simulink library "mag_vec_lib"  (R2016b)
settings: Solver=VariableStepAuto  StartTime=0.0  StopTime=10.0  RelTol=1e-3
undefined symbols (not defined in the file or in its folder): Earth, fsw_params, WGS84
libraries: aerolibtransform2 x2, dspmathops x1, aerolibgravity2 x1, YMDHMS_2_dec_year x1
settings Model: Creator=Taylor  LastModifiedBy=Taylor

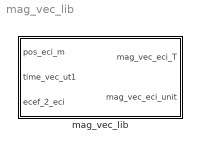
== system mag_vec_lib ==
  mag_vec_lib : Subsystem

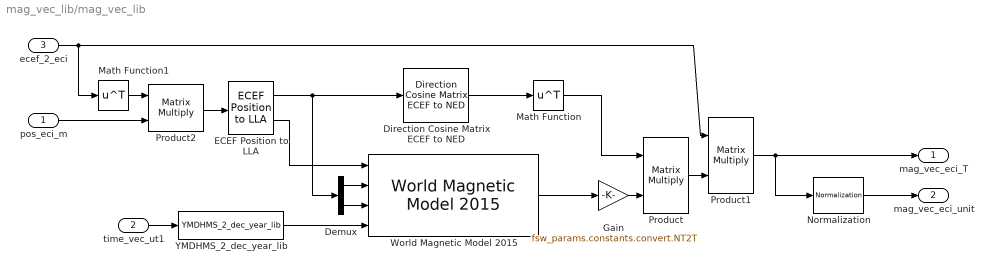
== system mag_vec_lib/mag_vec_lib ==
  pos_eci_m : Inport
  time_vec_ut1 : Inport  Port=2
  ecef_2_eci : Inport  Port=3
  Demux : Demux  Outputs=2
  Direction Cosine Matrix ECEF to NED : aerolibtransform2/Direction Cosine Matrix ECEF to NED
  ECEF Position to LLA : aerolibtransform2/ECEF Position to LLA  units=Metric (MKS)  ptype=Earth (WGS84)  F=1/298.257223563  R=6378137
  Gain : Gain  Gain=fsw_params.constants.convert.NT2T
  Math Function : Math  Operator=transpose  SaturateOnIntegerOverflow=on
  Math Function1 : Math  Operator=transpose  SaturateOnIntegerOverflow=on
  Normalization : dspmathops/Normalization  NormType=2-norm  Bias=1e-10  NormOver=Each column  Dimension=1  outputDataTypeStr=Inherit: Same as product output  outputLastDataTypeStr=Inherit: Same as product output  outputMin=[]  outputMax=[]  accumDataTypeStr=Inherit: Same as product output  accumLastDataTypeStr=Inherit: Same as product output  roundingMode=Floor  overflowMode=off
  Product : Product  Multiplication=Matrix(*)
  Product1 : Product  Multiplication=Matrix(*)
  Product2 : Product  Multiplication=Matrix(*)
  World Magnetic Model 2015 : aerolibgravity2/World Magnetic Model 2015  units=Metric (MKS)  time_in=on  month=January  day=1  year=2015  action=Error  h_out=off  dec_out=off  inc_out=off  ti_out=off
  YMDHMS_2_dec_year_lib : YMDHMS_2_dec_year/YMDHMS_2_dec_year_lib
  mag_vec_eci_T : Outport
  mag_vec_eci_unit : Outport  Port=2
  wires:
  ECEF Position to LLA/1 -> Demux/1, Direction Cosine Matrix ECEF to NED/1
  ECEF Position to LLA/2 -> World Magnetic Model 2015/1
  pos_eci_m/1 -> Product2/2
  Gain/1 -> Product/2
  Direction Cosine Matrix ECEF to NED/1 -> Math Function/1
  Demux/1 -> World Magnetic Model 2015/2
  Demux/2 -> World Magnetic Model 2015/3
  Math Function/1 -> Product/1
  Product/1 -> Product1/2
  ecef_2_eci/1 -> Product1/1, Math Function1/1
  Product1/1 -> Normalization/1, mag_vec_eci_T/1
  Normalization/1 -> mag_vec_eci_unit/1
  YMDHMS_2_dec_year_lib/1 -> World Magnetic Model 2015/4
  time_vec_ut1/1 -> YMDHMS_2_dec_year_lib/1
  Math Function1/1 -> Product2/1
  Product2/1 -> ECEF Position to LLA/1
  World Magnetic Model 2015/1 -> Gain/1
